simulink model "SMIB_linearized"  (R2016b)
settings: Solver=VariableStepAuto  StartTime=0.0  StopTime=100  RelTol=1e-3
values from neighbouring files (symbols this model uses):
  D_gen = 2    [SMIB.m]
  k1 = 1/Delta*(iq_eq*(xq_p-xd_p)*(-r_line*cos(delta_eq)+(x_line+xq_p)*sin(delta_eq))+(eq_eq+(xq_p-xd_p)*id_eq)*((x_line+xd_p)*cos(delta_eq)+r_line*sin(delta_eq)))    [SMIB.m]
  k2 = iq_eq+1/Delta*((xq_p-xd_p)*(x_line+xq_p)*iq_eq+r_line*eq_eq+r_line*(xq_p-xd_p)*id_eq)    [SMIB.m]
  k3 = (1+(xd-xd_p)*(x_line+xq_p)/Delta)^-1    [SMIB.m]
  k4 = (xd-xd_p)/Delta*(-r_line*cos(delta_eq)+(x_line+xq_p)*sin(delta_eq))    [SMIB.m]
  k5 = 1/Delta*(vd_eq/vabs_eq*xq_p*((x_line+xd_p)*cos(delta_eq)+r_line*sin(delta_eq))-vq_eq/vabs_eq*xd_p*(-r_line*cos(delta_eq)+(x_line+xq_p)*sin(delta_eq)))    [SMIB.m]
  k6 = 1/Delta*(vd_eq/vabs_eq*xq_p*r_line+vq_eq/vabs_eq*xd_p*(x_line+xq_p))    [SMIB.m]
  KA = 30    [SMIB.m]
  M_gen = 8    [SMIB.m]
  TA = 0.2    [SMIB.m]
  Td = 6    [SMIB.m]
settings Model: Creator=dc  LastModifiedBy=dc

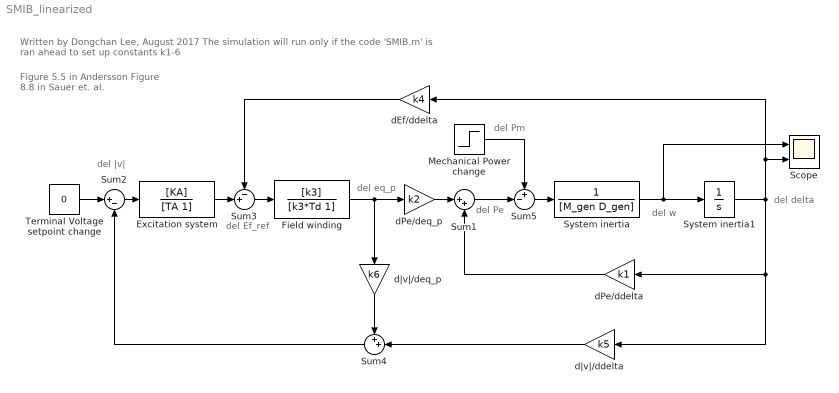
== system SMIB_linearized ==
  note: Written by Dongchan Lee, August 2017
      | The simulation will run only if the code 'SMIB.m' is ran ahead to set up constants k1-6
  note: Figure 5.5 in Andersson
      | Figure 8.8 in Sauer et. al.
  note: del |v|
  note: del delta
  note: del eq_p
  note: del Pm
  note: del Pe
  note: del w
  note: del Ef_ref
  Excitation system : TransferFcn  Numerator=[KA]  Denominator=[TA 1]
  Field winding : TransferFcn  Numerator=[k3]  Denominator=[k3*Td 1]
  Mechanical Power change : Step  SampleTime=0
  Scope : Scope  NumInputPorts=2
  Sum1 : Sum  Inputs=|++
  Sum2 : Sum  Inputs=|+-
  Sum3 : Sum  Inputs=-+|
  Sum4 : Sum  Inputs=++|
  Sum5 : Sum  Inputs=+-|
  System inertia : TransferFcn  Denominator=[M_gen D_gen]
  System inertia1 : TransferFcn  Denominator=[1 0]
  Terminal Voltage setpoint change : Constant  Value=0
  dEf/ddelta : Gain  Gain=k4
  dPe/ddelta : Gain  Gain=k1
  dPe/deq_p : Gain  Gain=k2
  d|v|/ddelta : Gain  Gain=k5
  d|v|/deq_p : Gain  Gain=k6
  wires:
  Mechanical Power change/1 -> Sum5/1
  Sum5/1 -> System inertia/1
  System inertia/1 -> System inertia1/1, Scope/1
  System inertia1/1 -> d|v|/ddelta/1, dPe/ddelta/1, dEf/ddelta/1, Scope/2
  Sum1/1 -> Sum5/2
  dPe/ddelta/1 -> Sum1/2
  Field winding/1 -> d|v|/deq_p/1, dPe/deq_p/1
  Sum3/1 -> Field winding/1
  Sum2/1 -> Excitation system/1
  dEf/ddelta/1 -> Sum3/1
  d|v|/deq_p/1 -> Sum4/1
  d|v|/ddelta/1 -> Sum4/2
  Sum4/1 -> Sum2/2
  Terminal Voltage setpoint change/1 -> Sum2/1
  dPe/deq_p/1 -> Sum1/1
  Excitation system/1 -> Sum3/2
